simulink model "cascade"  (R2020a)
settings: Solver=VariableStepAuto  StartTime=0.0  StopTime=200  RelTol=1e-3
libraries: simulink x15
settings Model: Creator=Noel  LastModifiedBy=Noel

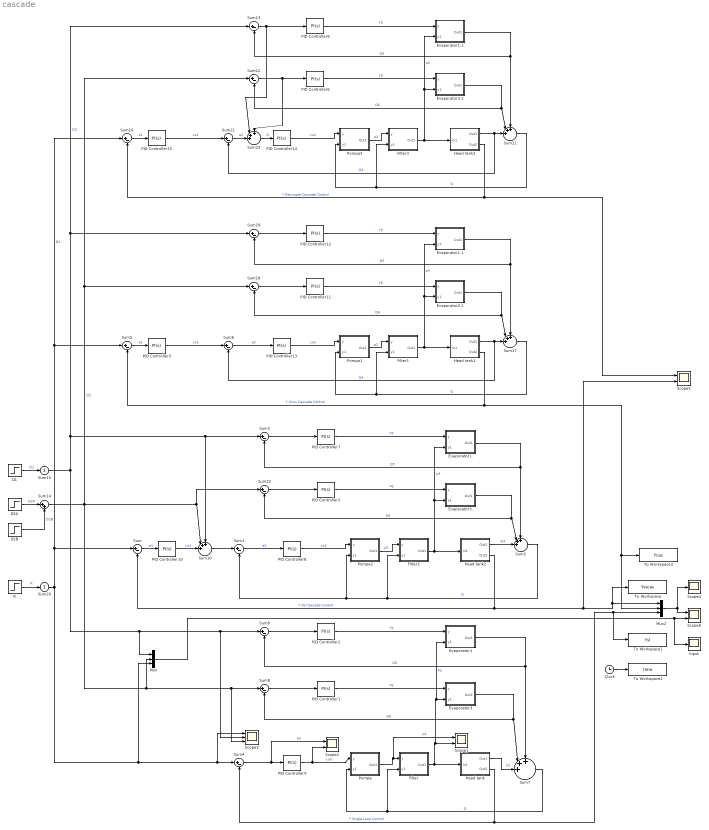
== system cascade ==
  Clock : Clock
  D1 : Step  Time=50  SampleTime=0
  D2A : Step  Time=100  After=0.5  SampleTime=0
  D2B : Step  Time=150  After=0.5  SampleTime=0
  Evaporator1 : Subsystem
  Evaporator1. : Subsystem
  Evaporator1.1 : Subsystem
  Evaporator1.2 : Subsystem
  Evaporator3 : Subsystem
  Evaporator3. : Subsystem
  Evaporator3.1 : Subsystem
  Evaporator3.2 : Subsystem
  Filter : Subsystem
  Filter1 : Subsystem
  Filter2 : Subsystem
  Filter3 : Subsystem
  Head tank : Subsystem
  Head tank1 : Subsystem
  Head tank2 : Subsystem
  Head tank3 : Subsystem
  Input : Scope
  Mux : Mux  Inputs=3
  Mux2 : Mux  Inputs=3
  PID Controller{1..2,5..7,9,11..12} (8 alike) : simulink/Continuous/PID Controller  Controller=PI  Form=Parallel  TimeDomain=Continuous-time  UseExternalTs=off  SampleTime=-1  IntegratorMethod=Forward Euler  FilterMethod=Forward Euler  ControllerParametersSource=internal  P=1.23205080756888  I=1.24401693585629  D=0.0542671517574869  UseFilter=on  N=20.3539436942361  TunerSelectOption=Transfer Function Based (PID Tuner App)  InitialConditionSource=internal  InitialConditionForIntegrator=0  InitialConditionForFilter=0  DifferentiatorICPrevScaledInput=0  ExternalReset=none  TrackingMode=off  Kt=1  LimitOutput=off  UpperSaturationLimit=inf  LowerSaturationLimit=-inf  LinearizeAsGain=on  AntiWindupMode=none  Kb=1  POutMin=[]  POutMax=[]  IOutMin=[]  IOutMax=[]  DOutMin=[]  DOutMax=[]  NOutMin=[]  NOutMax=[]  SumOutMin=[]  SumOutMax=[]  SaturationOutMin=[]  SaturationOutMax=[]  PParamMin=[]  PParamMax=[]  IParamMin=[]  IParamMax=[]  DParamMin=[]  DParamMax=[]  NParamMin=[]  NParamMax=[]  KbParamMin=[]  KbParamMax=[]  KtParamMin=[]  KtParamMax=[]  KbOutMin=[]  KbOutMax=[]  KtOutMin=[]  KtOutMax=[]  IntegratorOutMin=[]  IntegratorOutMax=[]  FilterOutMin=[]  FilterOutMax=[]  SumI1OutMin=[]  SumI1OutMax=[]  SumI2OutMin=[]  SumI2OutMax=[]  SumI3OutMin=[]  SumI3OutMax=[]  SumI4OutMin=[]  SumI4OutMax=[]  SumDOutMin=[]  SumDOutMax=[]  DifferentiatorOutMin=[]  DifferentiatorOutMax=[]  FilterDiffOutCoefMin=[]  FilterDiffOutCoefMax=[]  ReciprocalOutMin=[]  ReciprocalOutMax=[]  SumDenOutMin=[]  SumDenOutMax=[]  SumNumOutMin=[]  SumNumOutMax=[]  DivideOutMin=[]  DivideOutMax=[]  UdiffTsProdOutMin=[]  UdiffTsProdOutMax=[]  NTsProdOutMin=[]  NTsProdOutMax=[]  UintegralTsProdOutMin=[]  UintegralTsProdOutMax=[]  UngainTsProdOutMin=[]  UngainTsProdOutMax=[]  IntegratorContinuousStateAttributes=''  IntegratorStateMustResolveToSignalObject=off  IntegratorRTWStateStorageClass=Auto  FilterContinuousStateAttributes=''  FilterStateMustResolveToSignalObject=off  FilterRTWStateStorageClass=Auto  ParallelPVariant=InternalParameters  IdealPVariant=Disabled  IVariant=InternalParameters  DVariant=Disabled  IntegratorVariant=Continuous  SatVariant=Disabled  AWVariant=Passthrough  PCopyVariant=Disabled  TRVariant=Disabled  FdbkBlocksVariant=Forward  IdealPFdbkVariant=Disabled  SatFdbkVariant=Disabled  DerivativeFilterVariant=Disabled  NVariant=Disabled  NCopyVariant=Disabled_SignalSpec  FilterICVariant=Disabled  IntegratorICVariant=InternalICs  ExternalResetVariant=Disabled  TRSumVariant=Passthrough  SumFdbkVariant=Disabled  SumVariant=Sum_PI  TsampFilterVariant=InternalTs  TsampNgainVariant=Passthrough  TsampIntegralVariant=Passthrough
  PID Controller10 : simulink/Continuous/PID Controller  Controller=PI  Form=Parallel  TimeDomain=Continuous-time  UseExternalTs=off  SampleTime=-1  IntegratorMethod=Forward Euler  FilterMethod=Forward Euler  ControllerParametersSource=internal  P=0.968672981821934  I=0.0970699899095717  D=0  UseFilter=on  N=100  TunerSelectOption=Transfer Function Based (PID Tuner App)  InitialConditionSource=internal  InitialConditionForIntegrator=0  InitialConditionForFilter=0  DifferentiatorICPrevScaledInput=0  ExternalReset=none  TrackingMode=off  Kt=1  LimitOutput=off  UpperSaturationLimit=inf  LowerSaturationLimit=-inf  LinearizeAsGain=on  AntiWindupMode=none  Kb=1  POutMin=[]  POutMax=[]  IOutMin=[]  IOutMax=[]  DOutMin=[]  DOutMax=[]  NOutMin=[]  NOutMax=[]  SumOutMin=[]  SumOutMax=[]  SaturationOutMin=[]  SaturationOutMax=[]  PParamMin=[]  PParamMax=[]  IParamMin=[]  IParamMax=[]  DParamMin=[]  DParamMax=[]  NParamMin=[]  NParamMax=[]  KbParamMin=[]  KbParamMax=[]  KtParamMin=[]  KtParamMax=[]  KbOutMin=[]  KbOutMax=[]  KtOutMin=[]  KtOutMax=[]  IntegratorOutMin=[]  IntegratorOutMax=[]  FilterOutMin=[]  FilterOutMax=[]  SumI1OutMin=[]  SumI1OutMax=[]  SumI2OutMin=[]  SumI2OutMax=[]  SumI3OutMin=[]  SumI3OutMax=[]  SumI4OutMin=[]  SumI4OutMax=[]  SumDOutMin=[]  SumDOutMax=[]  DifferentiatorOutMin=[]  DifferentiatorOutMax=[]  FilterDiffOutCoefMin=[]  FilterDiffOutCoefMax=[]  ReciprocalOutMin=[]  ReciprocalOutMax=[]  SumDenOutMin=[]  SumDenOutMax=[]  SumNumOutMin=[]  SumNumOutMax=[]  DivideOutMin=[]  DivideOutMax=[]  UdiffTsProdOutMin=[]  UdiffTsProdOutMax=[]  NTsProdOutMin=[]  NTsProdOutMax=[]  UintegralTsProdOutMin=[]  UintegralTsProdOutMax=[]  UngainTsProdOutMin=[]  UngainTsProdOutMax=[]  IntegratorContinuousStateAttributes=''  IntegratorStateMustResolveToSignalObject=off  IntegratorRTWStateStorageClass=Auto  FilterContinuousStateAttributes=''  FilterStateMustResolveToSignalObject=off  FilterRTWStateStorageClass=Auto  ParallelPVariant=InternalParameters  IdealPVariant=Disabled  IVariant=InternalParameters  DVariant=Disabled  IntegratorVariant=Continuous  SatVariant=Disabled  AWVariant=Passthrough  PCopyVariant=Disabled  TRVariant=Disabled  FdbkBlocksVariant=Forward  IdealPFdbkVariant=Disabled  SatFdbkVariant=Disabled  DerivativeFilterVariant=Disabled  NVariant=Disabled  NCopyVariant=Disabled_SignalSpec  FilterICVariant=Disabled  IntegratorICVariant=InternalICs  ExternalResetVariant=Disabled  TRSumVariant=Passthrough  SumFdbkVariant=Disabled  SumVariant=Sum_PI  TsampFilterVariant=InternalTs  TsampNgainVariant=Passthrough  TsampIntegralVariant=Passthrough
  PID Controller13 : simulink/Continuous/PID Controller  Controller=PI  Form=Parallel  TimeDomain=Continuous-time  UseExternalTs=off  SampleTime=-1  IntegratorMethod=Forward Euler  FilterMethod=Forward Euler  ControllerParametersSource=internal  P=0.322371975646573  I=0.351912338155997  D=0  UseFilter=on  N=100  TunerSelectOption=Transfer Function Based (PID Tuner App)  InitialConditionSource=internal  InitialConditionForIntegrator=0  InitialConditionForFilter=0  DifferentiatorICPrevScaledInput=0  ExternalReset=none  TrackingMode=off  Kt=1  LimitOutput=off  UpperSaturationLimit=inf  LowerSaturationLimit=-inf  LinearizeAsGain=on  AntiWindupMode=none  Kb=1  POutMin=[]  POutMax=[]  IOutMin=[]  IOutMax=[]  DOutMin=[]  DOutMax=[]  NOutMin=[]  NOutMax=[]  SumOutMin=[]  SumOutMax=[]  SaturationOutMin=[]  SaturationOutMax=[]  PParamMin=[]  PParamMax=[]  IParamMin=[]  IParamMax=[]  DParamMin=[]  DParamMax=[]  NParamMin=[]  NParamMax=[]  KbParamMin=[]  KbParamMax=[]  KtParamMin=[]  KtParamMax=[]  KbOutMin=[]  KbOutMax=[]  KtOutMin=[]  KtOutMax=[]  IntegratorOutMin=[]  IntegratorOutMax=[]  FilterOutMin=[]  FilterOutMax=[]  SumI1OutMin=[]  SumI1OutMax=[]  SumI2OutMin=[]  SumI2OutMax=[]  SumI3OutMin=[]  SumI3OutMax=[]  SumI4OutMin=[]  SumI4OutMax=[]  SumDOutMin=[]  SumDOutMax=[]  DifferentiatorOutMin=[]  DifferentiatorOutMax=[]  FilterDiffOutCoefMin=[]  FilterDiffOutCoefMax=[]  ReciprocalOutMin=[]  ReciprocalOutMax=[]  SumDenOutMin=[]  SumDenOutMax=[]  SumNumOutMin=[]  SumNumOutMax=[]  DivideOutMin=[]  DivideOutMax=[]  UdiffTsProdOutMin=[]  UdiffTsProdOutMax=[]  NTsProdOutMin=[]  NTsProdOutMax=[]  UintegralTsProdOutMin=[]  UintegralTsProdOutMax=[]  UngainTsProdOutMin=[]  UngainTsProdOutMax=[]  IntegratorContinuousStateAttributes=''  IntegratorStateMustResolveToSignalObject=off  IntegratorRTWStateStorageClass=Auto  FilterContinuousStateAttributes=''  FilterStateMustResolveToSignalObject=off  FilterRTWStateStorageClass=Auto  ParallelPVariant=InternalParameters  IdealPVariant=Disabled  IVariant=InternalParameters  DVariant=Disabled  IntegratorVariant=Continuous  SatVariant=Disabled  AWVariant=Passthrough  PCopyVariant=Disabled  TRVariant=Disabled  FdbkBlocksVariant=Forward  IdealPFdbkVariant=Disabled  SatFdbkVariant=Disabled  DerivativeFilterVariant=Disabled  NVariant=Disabled  NCopyVariant=Disabled_SignalSpec  FilterICVariant=Disabled  IntegratorICVariant=InternalICs  ExternalResetVariant=Disabled  TRSumVariant=Passthrough  SumFdbkVariant=Disabled  SumVariant=Sum_PI  TsampFilterVariant=InternalTs  TsampNgainVariant=Passthrough  TsampIntegralVariant=Passthrough
  PID Controller14 : simulink/Continuous/PID Controller  Controller=PI  Form=Parallel  TimeDomain=Continuous-time  UseExternalTs=off  SampleTime=-1  IntegratorMethod=Forward Euler  FilterMethod=Forward Euler  ControllerParametersSource=internal  P=0.322371975646573  I=0.351912338155997  D=0  UseFilter=on  N=100  TunerSelectOption=Transfer Function Based (PID Tuner App)  InitialConditionSource=internal  InitialConditionForIntegrator=0  InitialConditionForFilter=0  DifferentiatorICPrevScaledInput=0  ExternalReset=none  TrackingMode=off  Kt=1  LimitOutput=off  UpperSaturationLimit=inf  LowerSaturationLimit=-inf  LinearizeAsGain=on  AntiWindupMode=none  Kb=1  POutMin=[]  POutMax=[]  IOutMin=[]  IOutMax=[]  DOutMin=[]  DOutMax=[]  NOutMin=[]  NOutMax=[]  SumOutMin=[]  SumOutMax=[]  SaturationOutMin=[]  SaturationOutMax=[]  PParamMin=[]  PParamMax=[]  IParamMin=[]  IParamMax=[]  DParamMin=[]  DParamMax=[]  NParamMin=[]  NParamMax=[]  KbParamMin=[]  KbParamMax=[]  KtParamMin=[]  KtParamMax=[]  KbOutMin=[]  KbOutMax=[]  KtOutMin=[]  KtOutMax=[]  IntegratorOutMin=[]  IntegratorOutMax=[]  FilterOutMin=[]  FilterOutMax=[]  SumI1OutMin=[]  SumI1OutMax=[]  SumI2OutMin=[]  SumI2OutMax=[]  SumI3OutMin=[]  SumI3OutMax=[]  SumI4OutMin=[]  SumI4OutMax=[]  SumDOutMin=[]  SumDOutMax=[]  DifferentiatorOutMin=[]  DifferentiatorOutMax=[]  FilterDiffOutCoefMin=[]  FilterDiffOutCoefMax=[]  ReciprocalOutMin=[]  ReciprocalOutMax=[]  SumDenOutMin=[]  SumDenOutMax=[]  SumNumOutMin=[]  SumNumOutMax=[]  DivideOutMin=[]  DivideOutMax=[]  UdiffTsProdOutMin=[]  UdiffTsProdOutMax=[]  NTsProdOutMin=[]  NTsProdOutMax=[]  UintegralTsProdOutMin=[]  UintegralTsProdOutMax=[]  UngainTsProdOutMin=[]  UngainTsProdOutMax=[]  IntegratorContinuousStateAttributes=''  IntegratorStateMustResolveToSignalObject=off  IntegratorRTWStateStorageClass=Auto  FilterContinuousStateAttributes=''  FilterStateMustResolveToSignalObject=off  FilterRTWStateStorageClass=Auto  ParallelPVariant=InternalParameters  IdealPVariant=Disabled  IVariant=InternalParameters  DVariant=Disabled  IntegratorVariant=Continuous  SatVariant=Disabled  AWVariant=Passthrough  PCopyVariant=Disabled  TRVariant=Disabled  FdbkBlocksVariant=Forward  IdealPFdbkVariant=Disabled  SatFdbkVariant=Disabled  DerivativeFilterVariant=Disabled  NVariant=Disabled  NCopyVariant=Disabled_SignalSpec  FilterICVariant=Disabled  IntegratorICVariant=InternalICs  ExternalResetVariant=Disabled  TRSumVariant=Passthrough  SumFdbkVariant=Disabled  SumVariant=Sum_PI  TsampFilterVariant=InternalTs  TsampNgainVariant=Passthrough  TsampIntegralVariant=Passthrough
  PID Controller15 : simulink/Continuous/PID Controller  Controller=PI  Form=Parallel  TimeDomain=Continuous-time  UseExternalTs=off  SampleTime=-1  IntegratorMethod=Forward Euler  FilterMethod=Forward Euler  ControllerParametersSource=internal  P=0.968672981821934  I=0.0970699899095717  D=0  UseFilter=on  N=100  TunerSelectOption=Transfer Function Based (PID Tuner App)  InitialConditionSource=internal  InitialConditionForIntegrator=0  InitialConditionForFilter=0  DifferentiatorICPrevScaledInput=0  ExternalReset=none  TrackingMode=off  Kt=1  LimitOutput=off  UpperSaturationLimit=inf  LowerSaturationLimit=-inf  LinearizeAsGain=on  AntiWindupMode=none  Kb=1  POutMin=[]  POutMax=[]  IOutMin=[]  IOutMax=[]  DOutMin=[]  DOutMax=[]  NOutMin=[]  NOutMax=[]  SumOutMin=[]  SumOutMax=[]  SaturationOutMin=[]  SaturationOutMax=[]  PParamMin=[]  PParamMax=[]  IParamMin=[]  IParamMax=[]  DParamMin=[]  DParamMax=[]  NParamMin=[]  NParamMax=[]  KbParamMin=[]  KbParamMax=[]  KtParamMin=[]  KtParamMax=[]  KbOutMin=[]  KbOutMax=[]  KtOutMin=[]  KtOutMax=[]  IntegratorOutMin=[]  IntegratorOutMax=[]  FilterOutMin=[]  FilterOutMax=[]  SumI1OutMin=[]  SumI1OutMax=[]  SumI2OutMin=[]  SumI2OutMax=[]  SumI3OutMin=[]  SumI3OutMax=[]  SumI4OutMin=[]  SumI4OutMax=[]  SumDOutMin=[]  SumDOutMax=[]  DifferentiatorOutMin=[]  DifferentiatorOutMax=[]  FilterDiffOutCoefMin=[]  FilterDiffOutCoefMax=[]  ReciprocalOutMin=[]  ReciprocalOutMax=[]  SumDenOutMin=[]  SumDenOutMax=[]  SumNumOutMin=[]  SumNumOutMax=[]  DivideOutMin=[]  DivideOutMax=[]  UdiffTsProdOutMin=[]  UdiffTsProdOutMax=[]  NTsProdOutMin=[]  NTsProdOutMax=[]  UintegralTsProdOutMin=[]  UintegralTsProdOutMax=[]  UngainTsProdOutMin=[]  UngainTsProdOutMax=[]  IntegratorContinuousStateAttributes=''  IntegratorStateMustResolveToSignalObject=off  IntegratorRTWStateStorageClass=Auto  FilterContinuousStateAttributes=''  FilterStateMustResolveToSignalObject=off  FilterRTWStateStorageClass=Auto  ParallelPVariant=InternalParameters  IdealPVariant=Disabled  IVariant=InternalParameters  DVariant=Disabled  IntegratorVariant=Continuous  SatVariant=Disabled  AWVariant=Passthrough  PCopyVariant=Disabled  TRVariant=Disabled  FdbkBlocksVariant=Forward  IdealPFdbkVariant=Disabled  SatFdbkVariant=Disabled  DerivativeFilterVariant=Disabled  NVariant=Disabled  NCopyVariant=Disabled_SignalSpec  FilterICVariant=Disabled  IntegratorICVariant=InternalICs  ExternalResetVariant=Disabled  TRSumVariant=Passthrough  SumFdbkVariant=Disabled  SumVariant=Sum_PI  TsampFilterVariant=InternalTs  TsampNgainVariant=Passthrough  TsampIntegralVariant=Passthrough
  PID Controller3 : simulink/Continuous/PID Controller  Controller=PI  Form=Parallel  TimeDomain=Continuous-time  UseExternalTs=off  SampleTime=-1  IntegratorMethod=Forward Euler  FilterMethod=Forward Euler  ControllerParametersSource=internal  P=0.968672981821934  I=0.0970699899095717  D=0  UseFilter=on  N=100  TunerSelectOption=Transfer Function Based (PID Tuner App)  InitialConditionSource=internal  InitialConditionForIntegrator=0  InitialConditionForFilter=0  DifferentiatorICPrevScaledInput=0  ExternalReset=none  TrackingMode=off  Kt=1  LimitOutput=off  UpperSaturationLimit=inf  LowerSaturationLimit=-inf  LinearizeAsGain=on  AntiWindupMode=none  Kb=1  POutMin=[]  POutMax=[]  IOutMin=[]  IOutMax=[]  DOutMin=[]  DOutMax=[]  NOutMin=[]  NOutMax=[]  SumOutMin=[]  SumOutMax=[]  SaturationOutMin=[]  SaturationOutMax=[]  PParamMin=[]  PParamMax=[]  IParamMin=[]  IParamMax=[]  DParamMin=[]  DParamMax=[]  NParamMin=[]  NParamMax=[]  KbParamMin=[]  KbParamMax=[]  KtParamMin=[]  KtParamMax=[]  KbOutMin=[]  KbOutMax=[]  KtOutMin=[]  KtOutMax=[]  IntegratorOutMin=[]  IntegratorOutMax=[]  FilterOutMin=[]  FilterOutMax=[]  SumI1OutMin=[]  SumI1OutMax=[]  SumI2OutMin=[]  SumI2OutMax=[]  SumI3OutMin=[]  SumI3OutMax=[]  SumI4OutMin=[]  SumI4OutMax=[]  SumDOutMin=[]  SumDOutMax=[]  DifferentiatorOutMin=[]  DifferentiatorOutMax=[]  FilterDiffOutCoefMin=[]  FilterDiffOutCoefMax=[]  ReciprocalOutMin=[]  ReciprocalOutMax=[]  SumDenOutMin=[]  SumDenOutMax=[]  SumNumOutMin=[]  SumNumOutMax=[]  DivideOutMin=[]  DivideOutMax=[]  UdiffTsProdOutMin=[]  UdiffTsProdOutMax=[]  NTsProdOutMin=[]  NTsProdOutMax=[]  UintegralTsProdOutMin=[]  UintegralTsProdOutMax=[]  UngainTsProdOutMin=[]  UngainTsProdOutMax=[]  IntegratorContinuousStateAttributes=''  IntegratorStateMustResolveToSignalObject=off  IntegratorRTWStateStorageClass=Auto  FilterContinuousStateAttributes=''  FilterStateMustResolveToSignalObject=off  FilterRTWStateStorageClass=Auto  ParallelPVariant=InternalParameters  IdealPVariant=Disabled  IVariant=InternalParameters  DVariant=Disabled  IntegratorVariant=Continuous  SatVariant=Disabled  AWVariant=Passthrough  PCopyVariant=Disabled  TRVariant=Disabled  FdbkBlocksVariant=Forward  IdealPFdbkVariant=Disabled  SatFdbkVariant=Disabled  DerivativeFilterVariant=Disabled  NVariant=Disabled  NCopyVariant=Disabled_SignalSpec  FilterICVariant=Disabled  IntegratorICVariant=InternalICs  ExternalResetVariant=Disabled  TRSumVariant=Passthrough  SumFdbkVariant=Disabled  SumVariant=Sum_PI  TsampFilterVariant=InternalTs  TsampNgainVariant=Passthrough  TsampIntegralVariant=Passthrough
  PID Controller4 : simulink/Continuous/PID Controller  Controller=PI  Form=Parallel  TimeDomain=Continuous-time  UseExternalTs=off  SampleTime=-1  IntegratorMethod=Forward Euler  FilterMethod=Forward Euler  ControllerParametersSource=internal  P=1.22767766587212  I=0.156528896652304  D=0  UseFilter=on  N=100  TunerSelectOption=Transfer Function Based (PID Tuner App)  InitialConditionSource=internal  InitialConditionForIntegrator=0  InitialConditionForFilter=0  DifferentiatorICPrevScaledInput=0  ExternalReset=none  TrackingMode=off  Kt=1  LimitOutput=off  UpperSaturationLimit=inf  LowerSaturationLimit=-inf  LinearizeAsGain=on  AntiWindupMode=none  Kb=1  POutMin=[]  POutMax=[]  IOutMin=[]  IOutMax=[]  DOutMin=[]  DOutMax=[]  NOutMin=[]  NOutMax=[]  SumOutMin=[]  SumOutMax=[]  SaturationOutMin=[]  SaturationOutMax=[]  PParamMin=[]  PParamMax=[]  IParamMin=[]  IParamMax=[]  DParamMin=[]  DParamMax=[]  NParamMin=[]  NParamMax=[]  KbParamMin=[]  KbParamMax=[]  KtParamMin=[]  KtParamMax=[]  KbOutMin=[]  KbOutMax=[]  KtOutMin=[]  KtOutMax=[]  IntegratorOutMin=[]  IntegratorOutMax=[]  FilterOutMin=[]  FilterOutMax=[]  SumI1OutMin=[]  SumI1OutMax=[]  SumI2OutMin=[]  SumI2OutMax=[]  SumI3OutMin=[]  SumI3OutMax=[]  SumI4OutMin=[]  SumI4OutMax=[]  SumDOutMin=[]  SumDOutMax=[]  DifferentiatorOutMin=[]  DifferentiatorOutMax=[]  FilterDiffOutCoefMin=[]  FilterDiffOutCoefMax=[]  ReciprocalOutMin=[]  ReciprocalOutMax=[]  SumDenOutMin=[]  SumDenOutMax=[]  SumNumOutMin=[]  SumNumOutMax=[]  DivideOutMin=[]  DivideOutMax=[]  UdiffTsProdOutMin=[]  UdiffTsProdOutMax=[]  NTsProdOutMin=[]  NTsProdOutMax=[]  UintegralTsProdOutMin=[]  UintegralTsProdOutMax=[]  UngainTsProdOutMin=[]  UngainTsProdOutMax=[]  IntegratorContinuousStateAttributes=''  IntegratorStateMustResolveToSignalObject=off  IntegratorRTWStateStorageClass=Auto  FilterContinuousStateAttributes=''  FilterStateMustResolveToSignalObject=off  FilterRTWStateStorageClass=Auto  ParallelPVariant=InternalParameters  IdealPVariant=Disabled  IVariant=InternalParameters  DVariant=Disabled  IntegratorVariant=Continuous  SatVariant=Disabled  AWVariant=Passthrough  PCopyVariant=Disabled  TRVariant=Disabled  FdbkBlocksVariant=Forward  IdealPFdbkVariant=Disabled  SatFdbkVariant=Disabled  DerivativeFilterVariant=Disabled  NVariant=Disabled  NCopyVariant=Disabled_SignalSpec  FilterICVariant=Disabled  IntegratorICVariant=InternalICs  ExternalResetVariant=Disabled  TRSumVariant=Passthrough  SumFdbkVariant=Disabled  SumVariant=Sum_PI  TsampFilterVariant=InternalTs  TsampNgainVariant=Passthrough  TsampIntegralVariant=Passthrough
  PID Controller8 : simulink/Continuous/PID Controller  Controller=PI  Form=Parallel  TimeDomain=Continuous-time  UseExternalTs=off  SampleTime=-1  IntegratorMethod=Forward Euler  FilterMethod=Forward Euler  ControllerParametersSource=internal  P=0.322371975646573  I=0.351912338155997  D=0  UseFilter=on  N=100  TunerSelectOption=Transfer Function Based (PID Tuner App)  InitialConditionSource=internal  InitialConditionForIntegrator=0  InitialConditionForFilter=0  DifferentiatorICPrevScaledInput=0  ExternalReset=none  TrackingMode=off  Kt=1  LimitOutput=off  UpperSaturationLimit=inf  LowerSaturationLimit=-inf  LinearizeAsGain=on  AntiWindupMode=none  Kb=1  POutMin=[]  POutMax=[]  IOutMin=[]  IOutMax=[]  DOutMin=[]  DOutMax=[]  NOutMin=[]  NOutMax=[]  SumOutMin=[]  SumOutMax=[]  SaturationOutMin=[]  SaturationOutMax=[]  PParamMin=[]  PParamMax=[]  IParamMin=[]  IParamMax=[]  DParamMin=[]  DParamMax=[]  NParamMin=[]  NParamMax=[]  KbParamMin=[]  KbParamMax=[]  KtParamMin=[]  KtParamMax=[]  KbOutMin=[]  KbOutMax=[]  KtOutMin=[]  KtOutMax=[]  IntegratorOutMin=[]  IntegratorOutMax=[]  FilterOutMin=[]  FilterOutMax=[]  SumI1OutMin=[]  SumI1OutMax=[]  SumI2OutMin=[]  SumI2OutMax=[]  SumI3OutMin=[]  SumI3OutMax=[]  SumI4OutMin=[]  SumI4OutMax=[]  SumDOutMin=[]  SumDOutMax=[]  DifferentiatorOutMin=[]  DifferentiatorOutMax=[]  FilterDiffOutCoefMin=[]  FilterDiffOutCoefMax=[]  ReciprocalOutMin=[]  ReciprocalOutMax=[]  SumDenOutMin=[]  SumDenOutMax=[]  SumNumOutMin=[]  SumNumOutMax=[]  DivideOutMin=[]  DivideOutMax=[]  UdiffTsProdOutMin=[]  UdiffTsProdOutMax=[]  NTsProdOutMin=[]  NTsProdOutMax=[]  UintegralTsProdOutMin=[]  UintegralTsProdOutMax=[]  UngainTsProdOutMin=[]  UngainTsProdOutMax=[]  IntegratorContinuousStateAttributes=''  IntegratorStateMustResolveToSignalObject=off  IntegratorRTWStateStorageClass=Auto  FilterContinuousStateAttributes=''  FilterStateMustResolveToSignalObject=off  FilterRTWStateStorageClass=Auto  ParallelPVariant=InternalParameters  IdealPVariant=Disabled  IVariant=InternalParameters  DVariant=Disabled  IntegratorVariant=Continuous  SatVariant=Disabled  AWVariant=Passthrough  PCopyVariant=Disabled  TRVariant=Disabled  FdbkBlocksVariant=Forward  IdealPFdbkVariant=Disabled  SatFdbkVariant=Disabled  DerivativeFilterVariant=Disabled  NVariant=Disabled  NCopyVariant=Disabled_SignalSpec  FilterICVariant=Disabled  IntegratorICVariant=InternalICs  ExternalResetVariant=Disabled  TRSumVariant=Passthrough  SumFdbkVariant=Disabled  SumVariant=Sum_PI  TsampFilterVariant=InternalTs  TsampNgainVariant=Passthrough  TsampIntegralVariant=Passthrough
  Pompa : Subsystem
  Pompa1 : Subsystem
  Pompa2 : Subsystem
  Pompa3 : Subsystem
  R : Step  Time=0  SampleTime=0
  Scope{1..2,5..6} (4 alike) : Scope  NumInputPorts=2
  Scope3 : Scope  NumInputPorts=3
  Scope4 : Scope
  Sum{,1,3..6,8..9,12..13,16,18..19,21..22} (15 alike) : Sum  Inputs=|+-
  Sum{2,7,10..11,17,23} (6 alike) : Sum  Inputs=+++||
  Sum14 : Sum  Inputs=|++
  Sum15 : Sum  Inputs=+
  Sum20 : Sum  Inputs=+
  To Workspace : ToWorkspace  VariableName=Ysscas  SaveFormat=Timeseries  SampleTime=-1
  To Workspace1 : ToWorkspace  VariableName=Ysl  SaveFormat=Timeseries  SampleTime=-1
  To Workspace2 : ToWorkspace  VariableName=time  SaveFormat=Timeseries  SampleTime=-1
  To Workspace3 : ToWorkspace  VariableName=Ycas  SaveFormat=Timeseries  SampleTime=-1
  wires:
  Pompa2/1(Out1) -> Filter2/1(y)  "p2"
  PID Controller5/1 -> Evaporator3./1(y)  "Y6"
  Sum22/1 -> PID Controller5/1
  PID Controller7/1 -> Evaporator1./1(y)  "Y5"
  Head tank2/1(Out1) -> Sum2/3  "Q4"
  Sum3/1 -> PID Controller7/1
  PID Controller10/1 -> Sum10/3  "co1"
  Head tank2/2(Out2) -> Sum/2, Scope5/2, Mux2/1, To Workspace/1  "Y SS Cascade Control"
  PID Controller8/1 -> Pompa2/1(y)  "co2"
  Sum/1 -> PID Controller10/1  "e1"
  Sum2/1 -> Filter2/2(y1), Pompa2/2(y1), Sum1/2  "Q"
  PID Controller2/1 -> Evaporator1/1(y)  "Y5"
  PID Controller1/1 -> Evaporator3/1(y)  "Y6"
  Sum8/1 -> PID Controller1/1
  Head tank/1(Out1) -> Sum7/3  "f0"
  Head tank/2(Out2) -> Sum4/2, Mux2/3, To Workspace1/1  "Y Single Loop Control"
  Sum4/1 -> PID Controller4/1, Scope2/1  "e3"
  Pompa/1(Out1) -> Scope1/1, Filter/1(y)  "p2"
  PID Controller4/1 -> Pompa/1(y), Scope2/2  "co3"
  Sum7/1 -> Filter/2(y1), Pompa/2(y1)  "Q"
  Sum9/1 -> PID Controller2/1
  Filter2/1(Out1) -> Evaporator1./2(y1), Evaporator3./2(y1), Head tank2/1(In1)  "p3"
  Evaporator1./1(Out1) -> Sum2/1, Sum3/2  "Q5"
  Evaporator3./1(Out1) -> Sum22/2, Sum2/2  "Q6"
  Filter/1(Out1) -> Head tank/1(In1), Evaporator1/2(y1), Evaporator3/2(y1), Scope1/2  "P3"
  Evaporator1/1(Out1) -> Sum9/2, Sum7/1  "Q5"
  Evaporator3/1(Out1) -> Sum7/2, Sum8/2  "Q6"
  Clock/1 -> To Workspace2/1
  Mux/1 -> Input/1, Scope6/2
  Head tank1/2(Out2) -> Mux2/2, To Workspace3/1, Sum5/2  "Y Conv Cascade Control"
  Evaporator3.1/1(Out1) -> Sum17/2, Sum18/2  "Q6"
  Evaporator1.1/1(Out1) -> Sum17/1, Sum19/2  "Q5"
  Filter1/1(Out1) -> Evaporator1.1/2(y1), Evaporator3.1/2(y1), Head tank1/1(In1)  "p3"
  Sum5/1 -> PID Controller3/1  "e1"
  Sum18/1 -> PID Controller11/1
  Sum17/1 -> Filter1/2(y1), Pompa1/2(y1)  "Q"
  Head tank1/1(Out1) -> Sum6/2, Sum17/3  "Q4"
  PID Controller13/1 -> Pompa1/1(y)  "co2"
  Sum19/1 -> PID Controller12/1
  PID Controller11/1 -> Evaporator3.1/1(y)  "Y6"
  Sum6/1 -> PID Controller13/1  "e2"
  PID Controller12/1 -> Evaporator1.1/1(y)  "Y5"
  Pompa1/1(Out1) -> Filter1/1(y)  "p2"
  PID Controller3/1 -> Sum6/1  "co1"
  Sum1/1 -> PID Controller8/1  "e2"
  Mux2/1 -> Scope6/1, Scope4/1
  Sum10/1 -> Sum1/1
  D1/1 -> Sum15/1  "D1"
  D2A/1 -> Sum14/1  "D2A"
  D2B/1 -> Sum14/2  "D2B"
  R/1 -> Sum20/1  "R"
  Evaporator1.2/1(Out1) -> Sum11/1, Sum13/2  "Q5"
  Pompa3/1(Out1) -> Filter3/1(y)  "p2"
  PID Controller15/1 -> Sum21/1  "co1"
  Sum15/1 -> Sum13/1, Sum19/1, Sum3/1, Sum10/1, Mux/1, Scope3/2, Sum9/1  "D2"
  Evaporator3.2/1(Out1) -> Sum11/2, Sum12/2  "Q6"
  PID Controller14/1 -> Pompa3/1(y)  "co2"
  PID Controller9/1 -> Evaporator1.2/1(y)  "Y5"
  Sum20/1 -> Mux/3, Scope3/1, Sum4/1, Sum/1, Sum16/1, Sum5/1  "D2"
  Sum11/1 -> Filter3/2(y1), Pompa3/2(y1)  "Q"
  Sum12/1 -> PID Controller6/1, Sum23/1
  Sum13/1 -> Sum23/2, PID Controller9/1
  Sum16/1 -> PID Controller15/1  "e1"
  Sum14/1 -> Sum10/2, Sum22/1, Sum12/1, Sum18/1, Mux/2, Scope3/3, Sum8/1  "D2"
  Filter3/1(Out1) -> Evaporator1.2/2(y1), Evaporator3.2/2(y1), Head tank3/1(In1)  "p3"
  Head tank3/1(Out1) -> Sum21/2, Sum11/3  "Q4"
  Head tank3/2(Out2) -> Scope5/1, Sum16/2  "Y Decouple Cascade Control"
  PID Controller6/1 -> Evaporator3.2/1(y)  "Y6"
  Sum21/1 -> Sum23/3  "e2"
  Sum23/1 -> PID Controller14/1  "Q"

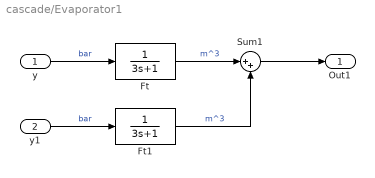
== system cascade/Evaporator1 ==
  y : Inport
  y1 : Inport  Port=2
  Ft : TransferFcn  Denominator=[3 1]
  Ft1 : TransferFcn  Denominator=[3 1]
  Sum1 : Sum  Inputs=|++
  Out1 : Outport
  wires:
  y/1 -> Ft/1  "bar"
  Ft/1 -> Sum1/1  "m^3"
  Sum1/1 -> Out1/1
  Ft1/1 -> Sum1/2  "m^3"
  y1/1 -> Ft1/1  "bar"

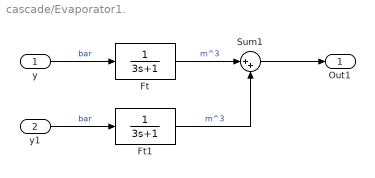
== system cascade/Evaporator1. ==
  y : Inport
  y1 : Inport  Port=2
  Ft : TransferFcn  Denominator=[3 1]
  Ft1 : TransferFcn  Denominator=[3 1]
  Sum1 : Sum  Inputs=|++
  Out1 : Outport
  wires:
  y/1 -> Ft/1  "bar"
  Ft/1 -> Sum1/1  "m^3"
  Sum1/1 -> Out1/1
  Ft1/1 -> Sum1/2  "m^3"
  y1/1 -> Ft1/1  "bar"

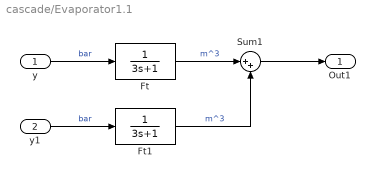
== system cascade/Evaporator1.1 ==
  y : Inport
  y1 : Inport  Port=2
  Ft : TransferFcn  Denominator=[3 1]
  Ft1 : TransferFcn  Denominator=[3 1]
  Sum1 : Sum  Inputs=|++
  Out1 : Outport
  wires:
  y/1 -> Ft/1  "bar"
  Ft/1 -> Sum1/1  "m^3"
  Sum1/1 -> Out1/1
  Ft1/1 -> Sum1/2  "m^3"
  y1/1 -> Ft1/1  "bar"

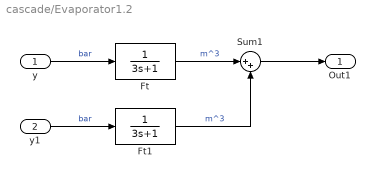
== system cascade/Evaporator1.2 ==
  y : Inport
  y1 : Inport  Port=2
  Ft : TransferFcn  Denominator=[3 1]
  Ft1 : TransferFcn  Denominator=[3 1]
  Sum1 : Sum  Inputs=|++
  Out1 : Outport
  wires:
  y/1 -> Ft/1  "bar"
  Ft/1 -> Sum1/1  "m^3"
  Sum1/1 -> Out1/1
  Ft1/1 -> Sum1/2  "m^3"
  y1/1 -> Ft1/1  "bar"

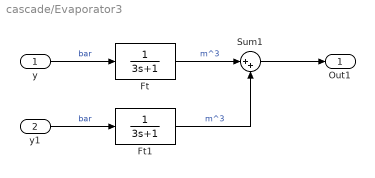
== system cascade/Evaporator3 ==
  y : Inport
  y1 : Inport  Port=2
  Ft : TransferFcn  Denominator=[3 1]
  Ft1 : TransferFcn  Denominator=[3 1]
  Sum1 : Sum  Inputs=|++
  Out1 : Outport
  wires:
  y/1 -> Ft/1  "bar"
  Ft/1 -> Sum1/1  "m^3"
  Sum1/1 -> Out1/1
  Ft1/1 -> Sum1/2  "m^3"
  y1/1 -> Ft1/1  "bar"

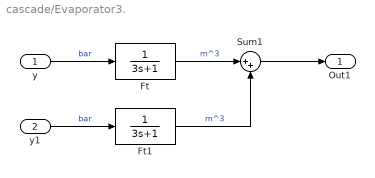
== system cascade/Evaporator3. ==
  y : Inport
  y1 : Inport  Port=2
  Ft : TransferFcn  Denominator=[3 1]
  Ft1 : TransferFcn  Denominator=[3 1]
  Sum1 : Sum  Inputs=|++
  Out1 : Outport
  wires:
  y/1 -> Ft/1  "bar"
  Ft/1 -> Sum1/1  "m^3"
  Sum1/1 -> Out1/1
  Ft1/1 -> Sum1/2  "m^3"
  y1/1 -> Ft1/1  "bar"

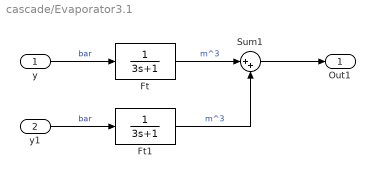
== system cascade/Evaporator3.1 ==
  y : Inport
  y1 : Inport  Port=2
  Ft : TransferFcn  Denominator=[3 1]
  Ft1 : TransferFcn  Denominator=[3 1]
  Sum1 : Sum  Inputs=|++
  Out1 : Outport
  wires:
  y/1 -> Ft/1  "bar"
  Ft/1 -> Sum1/1  "m^3"
  Sum1/1 -> Out1/1
  Ft1/1 -> Sum1/2  "m^3"
  y1/1 -> Ft1/1  "bar"

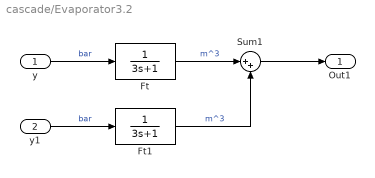
== system cascade/Evaporator3.2 ==
  y : Inport
  y1 : Inport  Port=2
  Ft : TransferFcn  Denominator=[3 1]
  Ft1 : TransferFcn  Denominator=[3 1]
  Sum1 : Sum  Inputs=|++
  Out1 : Outport
  wires:
  y/1 -> Ft/1  "bar"
  Ft/1 -> Sum1/1  "m^3"
  Sum1/1 -> Out1/1
  Ft1/1 -> Sum1/2  "m^3"
  y1/1 -> Ft1/1  "bar"

== system cascade/Filter ==
  y : Inport
  y1 : Inport  Port=2
  Ft : TransferFcn  Denominator=[1 1]
  Ft1 : TransferFcn  Numerator=[0.2]  Denominator=[1 1]
  Sum1 : Sum  Inputs=|+-
  Out1 : Outport
  wires:
  y/1 -> Ft/1  "bar"
  Ft/1 -> Sum1/1  "m^3"
  Sum1/1 -> Out1/1
  Ft1/1 -> Sum1/2  "m^3"
  y1/1 -> Ft1/1  "bar"

== system cascade/Filter1 ==
  y : Inport
  y1 : Inport  Port=2
  Ft : TransferFcn  Denominator=[1 1]
  Ft1 : TransferFcn  Numerator=[0.2]  Denominator=[1 1]
  Sum1 : Sum  Inputs=|+-
  Out1 : Outport
  wires:
  y/1 -> Ft/1  "bar"
  Ft/1 -> Sum1/1  "m^3"
  Sum1/1 -> Out1/1
  Ft1/1 -> Sum1/2  "m^3"
  y1/1 -> Ft1/1  "bar"

== system cascade/Filter2 ==
  y : Inport
  y1 : Inport  Port=2
  Ft : TransferFcn  Denominator=[1 1]
  Ft1 : TransferFcn  Numerator=[0.2]  Denominator=[1 1]
  Sum1 : Sum  Inputs=|+-
  Out1 : Outport
  wires:
  y/1 -> Ft/1  "bar"
  Ft/1 -> Sum1/1  "m^3"
  Sum1/1 -> Out1/1
  Ft1/1 -> Sum1/2  "m^3"
  y1/1 -> Ft1/1  "bar"

== system cascade/Filter3 ==
  y : Inport
  y1 : Inport  Port=2
  Ft : TransferFcn  Denominator=[1 1]
  Ft1 : TransferFcn  Numerator=[0.2]  Denominator=[1 1]
  Sum1 : Sum  Inputs=|+-
  Out1 : Outport
  wires:
  y/1 -> Ft/1  "bar"
  Ft/1 -> Sum1/1  "m^3"
  Sum1/1 -> Out1/1
  Ft1/1 -> Sum1/2  "m^3"
  y1/1 -> Ft1/1  "bar"

== system cascade/Head tank ==
  In1 : Inport
  Ft : TransferFcn  Denominator=[1 1]
  Ft1 : TransferFcn  Denominator=[10 1]
  Out1 : Outport
  Out2 : Outport  Port=2
  wires:
  Ft/1 -> Ft1/1, Out1/1  "m^3"
  In1/1 -> Ft/1
  Ft1/1 -> Out2/1  "m^3"

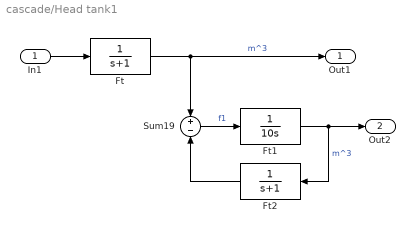
== system cascade/Head tank1 ==
  In1 : Inport
  Ft : TransferFcn  Denominator=[1 1]
  Ft1 : TransferFcn  Denominator=[10 0]
  Ft2 : TransferFcn  Denominator=[1 1]
  Sum19 : Sum  Inputs=+|-
  Out1 : Outport
  Out2 : Outport  Port=2
  wires:
  Ft/1 -> Sum19/1, Out1/1  "m^3"
  In1/1 -> Ft/1
  Ft1/1 -> Ft2/1, Out2/1  "m^3"
  Sum19/1 -> Ft1/1  "f1"
  Ft2/1 -> Sum19/2

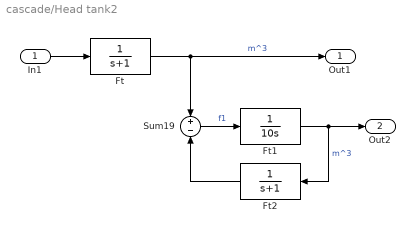
== system cascade/Head tank2 ==
  In1 : Inport
  Ft : TransferFcn  Denominator=[1 1]
  Ft1 : TransferFcn  Denominator=[10 0]
  Ft2 : TransferFcn  Denominator=[1 1]
  Sum19 : Sum  Inputs=+|-
  Out1 : Outport
  Out2 : Outport  Port=2
  wires:
  Ft/1 -> Sum19/1, Out1/1  "m^3"
  In1/1 -> Ft/1
  Ft1/1 -> Ft2/1, Out2/1  "m^3"
  Sum19/1 -> Ft1/1  "f1"
  Ft2/1 -> Sum19/2

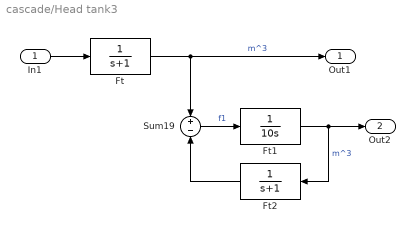
== system cascade/Head tank3 ==
  In1 : Inport
  Ft : TransferFcn  Denominator=[1 1]
  Ft1 : TransferFcn  Denominator=[10 0]
  Ft2 : TransferFcn  Denominator=[1 1]
  Sum19 : Sum  Inputs=+|-
  Out1 : Outport
  Out2 : Outport  Port=2
  wires:
  Ft/1 -> Sum19/1, Out1/1  "m^3"
  In1/1 -> Ft/1
  Ft1/1 -> Ft2/1, Out2/1  "m^3"
  Sum19/1 -> Ft1/1  "f1"
  Ft2/1 -> Sum19/2

== system cascade/Pompa ==
  y : Inport
  y1 : Inport  Port=2
  Ft : TransferFcn  Denominator=[1 1]
  Ft1 : TransferFcn  Numerator=[0.2]  Denominator=[1 1]
  Sum1 : Sum  Inputs=|+-
  Out1 : Outport
  wires:
  y/1 -> Ft/1  "bar"
  Ft/1 -> Sum1/1  "m^3"
  Sum1/1 -> Out1/1
  Ft1/1 -> Sum1/2  "m^3"
  y1/1 -> Ft1/1  "bar"

== system cascade/Pompa1 ==
  y : Inport
  y1 : Inport  Port=2
  Ft : TransferFcn  Denominator=[1 1]
  Ft1 : TransferFcn  Numerator=[0.2]  Denominator=[1 1]
  Sum1 : Sum  Inputs=|+-
  Out1 : Outport
  wires:
  y/1 -> Ft/1  "bar"
  Ft/1 -> Sum1/1  "m^3"
  Sum1/1 -> Out1/1
  Ft1/1 -> Sum1/2  "m^3"
  y1/1 -> Ft1/1  "bar"

== system cascade/Pompa2 ==
  y : Inport
  y1 : Inport  Port=2
  Ft : TransferFcn  Denominator=[1 1]
  Ft1 : TransferFcn  Numerator=[0.2]  Denominator=[1 1]
  Sum1 : Sum  Inputs=|+-
  Out1 : Outport
  wires:
  y/1 -> Ft/1  "bar"
  Ft/1 -> Sum1/1  "m^3"
  Sum1/1 -> Out1/1
  Ft1/1 -> Sum1/2  "m^3"
  y1/1 -> Ft1/1  "bar"

== system cascade/Pompa3 ==
  y : Inport
  y1 : Inport  Port=2
  Ft : TransferFcn  Denominator=[1 1]
  Ft1 : TransferFcn  Numerator=[0.2]  Denominator=[1 1]
  Sum1 : Sum  Inputs=|+-
  Out1 : Outport
  wires:
  y/1 -> Ft/1  "bar"
  Ft/1 -> Sum1/1  "m^3"
  Sum1/1 -> Out1/1
  Ft1/1 -> Sum1/2  "m^3"
  y1/1 -> Ft1/1  "bar"
